simulink model "ext"  (R2025b)
settings: Solver=VariableStepAuto  StartTime=0.0  StopTime=100  RelTol=1e-3
values from neighbouring files (symbols this model uses):
  Amplitude = 40    [Lab1_SSM.m]
  Ao = Ae-L*Ce    [Lab1_SSM.m]
  Beq = 1.9976e-6    (= 1.9976e-06)    [Lab1_SSM.m]
  Bo = [Be L]    [Lab1_SSM.m]
  Co = eye(5)    [Lab1_SSM.m]
  Cp = [1 0 0]    [Lab1_SSM.m]
  Do = zeros(5,2)    [Lab1_SSM.m]
  Jeq = 9.3937e-7    (= 9.3937e-07)    [Lab1_SSM.m]
  Req = mot.R + sens.curr.Rs    [Lab1_SSM.m]
  tau_sf = 0.005    [Lab1_SSM.m]
  Ts = 0.001    [Lab1_SSM.m]
  w0 = 2*pi/0.1    (= 62.8318530718)    [Lab1_SSM.m]
undefined symbols (not defined in the file or in its folder): c, daq, drv, gbox, mot, sens, SS
settings Model: Creator=Simone  LastModifiedBy=Simone

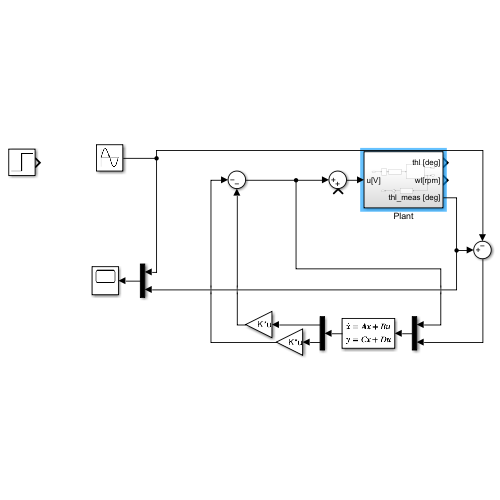
[thumbnail: Simulink's stored preview of the top-level diagram]
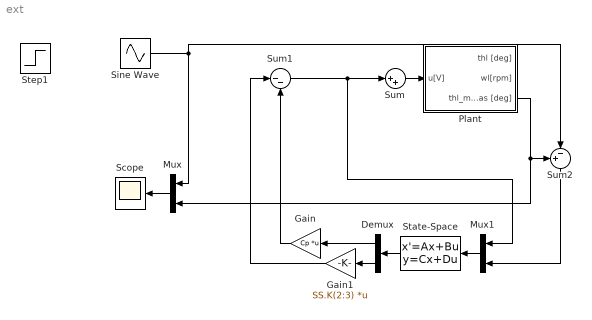
== system ext ==
  Demux : Demux  Outputs=2
  Gain : Gain  Gain=Cp  Multiplication=Matrix(K*u)
  Gain1 : Gain  Gain=SS.K(2:3)  Multiplication=Matrix(K*u)
  Mux : Mux  Inputs=2
  Mux1 : Mux  Inputs=2
  Plant : Subsystem
  Scope : Scope
      settings: ActiveDisplayYMinimum=-45.375067264512992  ActiveDisplayYMaximum=57.040290423093104
  Sine Wave : Sin  Amplitude=Amplitude  Frequency=w0  SampleTime=0
  State-Space : StateSpace  A=Ao  B=Bo  C=Co  D=Do  InitialCondition=0
  Step1 : Step  After=40  SampleTime=0
  Sum : Sum  Inputs=|++
  Sum1 : Sum  Inputs=|--
  Sum2 : Sum  Inputs=+-|
  wires:
  Mux/1 -> Scope/1
  Sine Wave/1 -> Mux/1, Sum2/2
  Mux1/1 -> State-Space/1
  State-Space/1 -> Demux/1
  Demux/2 -> Gain1/1
  Demux/1 -> Gain/1
  Sum/1 -> Plant/1(u[V])
  Sum1/1 -> Mux1/1, Sum/1
  Gain/1 -> Sum1/2
  Gain1/1 -> Sum1/1
  Sum2/1 -> Mux1/2
  Plant/3(thl_meas [deg]) -> Mux/2, Sum2/1

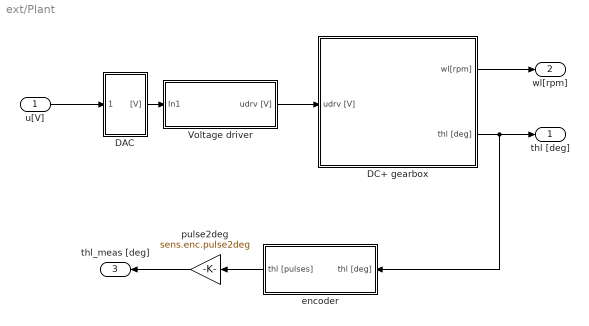
== system ext/Plant ==
  u[V] : Inport
  DAC : Subsystem
  DC+ gearbox : Subsystem
  Voltage driver : Subsystem
  encoder : Subsystem
  pulse2deg : Gain  Gain=sens.enc.pulse2deg
  thl [deg] : Outport
  wl[rpm] : Outport  Port=2
  thl_meas [deg] : Outport  Port=3
  wires:
  pulse2deg/1 -> thl_meas [deg]/1
  DC+ gearbox/2(thl [deg]) -> thl [deg]/1, encoder/1(thl [deg])
  Voltage driver/1(udrv [V]) -> DC+ gearbox/1(udrv [V])
  DC+ gearbox/1(wl[rpm]) -> wl[rpm]/1
  u[V]/1 -> DAC/1(In1)
  DAC/1("[V]") -> Voltage driver/1(In1)
  encoder/1(thl [pulses]) -> pulse2deg/1

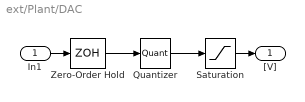
== system ext/Plant/DAC ==
  In1 : Inport
  Quantizer : Quantizer  QuantizationInterval=daq.dac.q
  Saturation : Saturate  UpperLimit=daq.dac.fs  LowerLimit=-daq.dac.fs
  Zero-Order Hold : ZeroOrderHold  SampleTime=Ts
  "[V]" : Outport
  wires:
  In1/1 -> Zero-Order Hold/1
  Zero-Order Hold/1 -> Quantizer/1
  Quantizer/1 -> Saturation/1
  Saturation/1 -> "[V]"/1

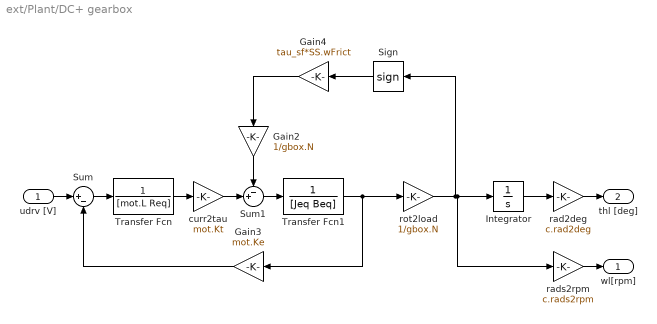
== system ext/Plant/DC+ gearbox ==
  udrv [V] : Inport
  Gain2 : Gain  Gain=1/gbox.N
  Gain3 : Gain  Gain=mot.Ke
  Gain4 : Gain  Gain=tau_sf*SS.wFrict
  Integrator : Integrator
  Sign : Signum  ZeroCross=off
  Sum : Sum  Inputs=|+-
  Sum1 : Sum  Inputs=-+|
  Transfer Fcn : TransferFcn  Denominator=[mot.L Req]
  Transfer Fcn1 : TransferFcn  Denominator=[Jeq Beq]
  curr2tau : Gain  Gain=mot.Kt
  rad2deg : Gain  Gain=c.rad2deg
  rads2rpm : Gain  Gain=c.rads2rpm
  rot2load : Gain  Gain=1/gbox.N
  wl[rpm] : Outport
  thl [deg] : Outport  Port=2
  wires:
  Sum/1 -> Transfer Fcn/1
  Gain2/1 -> Sum1/1
  Integrator/1 -> rad2deg/1
  Sign/1 -> Gain4/1
  udrv [V]/1 -> Sum/1
  Transfer Fcn1/1 -> Gain3/1, rot2load/1
  Gain3/1 -> Sum/2
  rot2load/1 -> Sign/1, rads2rpm/1, Integrator/1
  Sum1/1 -> Transfer Fcn1/1
  Gain4/1 -> Gain2/1
  Transfer Fcn/1 -> curr2tau/1
  rad2deg/1 -> thl [deg]/1
  curr2tau/1 -> Sum1/2
  rads2rpm/1 -> wl[rpm]/1

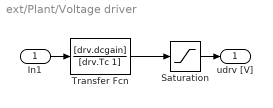
== system ext/Plant/Voltage driver ==
  In1 : Inport
  Saturation : Saturate  UpperLimit=drv.outmax  LowerLimit=-drv.outmax
  Transfer Fcn : TransferFcn  Numerator=[drv.dcgain]  Denominator=[drv.Tc 1]
  udrv [V] : Outport
  wires:
  Transfer Fcn/1 -> Saturation/1
  In1/1 -> Transfer Fcn/1
  Saturation/1 -> udrv [V]/1

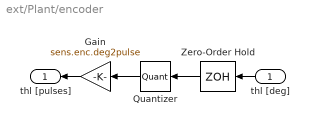
== system ext/Plant/encoder ==
  thl [deg] : Inport
  Gain : Gain  Gain=sens.enc.deg2pulse
  Quantizer : Quantizer  QuantizationInterval=daq.q
  Zero-Order Hold : ZeroOrderHold  SampleTime=Ts
  thl [pulses] : Outport
  wires:
  Zero-Order Hold/1 -> Quantizer/1
  Quantizer/1 -> Gain/1
  Gain/1 -> thl [pulses]/1
  thl [deg]/1 -> Zero-Order Hold/1
